simulink model "Regulator_1907_tests_2017a"  (R2017a)
settings: Solver=ode1  StartTime=0.0  StopTime=200  FixedStep=0.01  RelTol=1e-3
values from neighbouring files (symbols this model uses):
  Dist = 0.001    [my_test.m]
  Gain = 0.1    [my_test.m]
  Sat = 0.5    [my_test.m]
  Speed = 3    [my_test.m]
undefined symbols (not defined in the file or in its folder): DiscIntNeverNeededParam
settings Model: Creator=Dmitry  LastModifiedBy=makee
settings OptimizationCC: DefaultUnderspecifiedDataType=single

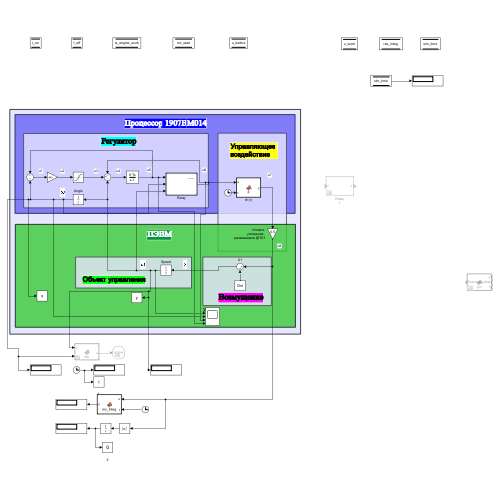
[thumbnail: Simulink's stored preview of the top-level diagram]
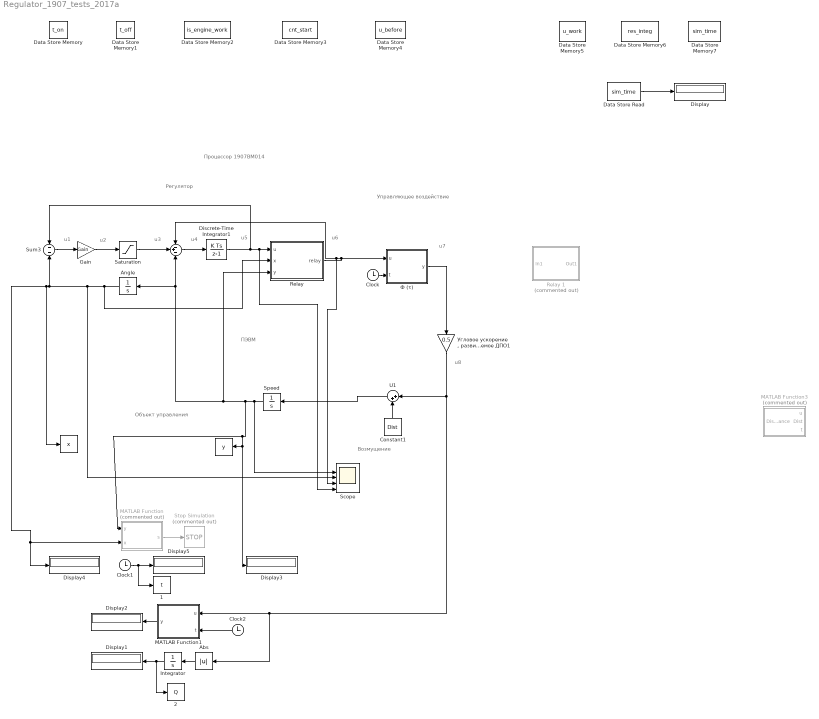
== system Regulator_1907_tests_2017a ==
  note: u8
  note: u7
  note: u6
  note: u5
  note: u4
  note: u3
  note: u2
  note: u1
  note: Объект управления
  note: Управляющее
      | воздействие
  note: Регулятор
  note: Возмущение
  note: ПЭВМ
  note: Процессор 1907ВM014
  " " : ToWorkspace  VariableName=y  SampleTime=-1
  " " : Sum  Inputs=-+-
  " " : ToWorkspace  VariableName=x  SampleTime=-1
  " 1" : ToWorkspace  VariableName=t  SampleTime=-1
  " 2" : ToWorkspace  VariableName=Q  SampleTime=-1
  Abs : Abs
  Angle : Integrator  AbsoluteTolerance=-1
  Clock : Clock
  Clock1 : Clock
  Clock2 : Clock
  Constant1 : Constant  Value=Dist  SampleTime=-1
  Data Store Memory : DataStoreMemory  DataStoreName=t_on  ReadBeforeWriteMsg=warning  WriteAfterWriteMsg=warning  WriteAfterReadMsg=warning  ShowAdditionalParam=off  OutDataTypeStr=double
  Data Store Memory1 : DataStoreMemory  DataStoreName=t_off  ReadBeforeWriteMsg=warning  WriteAfterWriteMsg=warning  WriteAfterReadMsg=warning  ShowAdditionalParam=off  OutDataTypeStr=double
  Data Store Memory2 : DataStoreMemory  DataStoreName=is_engine_work  ReadBeforeWriteMsg=warning  WriteAfterWriteMsg=warning  WriteAfterReadMsg=warning  ShowAdditionalParam=off  OutDataTypeStr=boolean
  Data Store Memory3 : DataStoreMemory  DataStoreName=cnt_start  ReadBeforeWriteMsg=warning  WriteAfterWriteMsg=warning  WriteAfterReadMsg=warning  ShowAdditionalParam=off  OutDataTypeStr=int8
  Data Store Memory4 : DataStoreMemory  DataStoreName=u_before  ReadBeforeWriteMsg=warning  WriteAfterWriteMsg=warning  WriteAfterReadMsg=warning  ShowAdditionalParam=off  OutDataTypeStr=double
  Data Store Memory5 : DataStoreMemory  DataStoreName=u_work  ReadBeforeWriteMsg=warning  WriteAfterWriteMsg=warning  WriteAfterReadMsg=warning  ShowAdditionalParam=off  OutDataTypeStr=double
  Data Store Memory6 : DataStoreMemory  DataStoreName=res_integ  ReadBeforeWriteMsg=warning  WriteAfterWriteMsg=warning  WriteAfterReadMsg=warning  ShowAdditionalParam=off  OutDataTypeStr=double
  Data Store Memory7 : DataStoreMemory  DataStoreName=sim_time  ReadBeforeWriteMsg=warning  WriteAfterWriteMsg=warning  WriteAfterReadMsg=warning  InitialValue=200  ShowAdditionalParam=off  OutDataTypeStr=double
  Data Store Read : DataStoreRead  DataStoreName=sim_time
  Discrete-Time Integrator1 : DiscreteIntegrator  InitialConditionSetting=State (most efficient)  SampleTime=-1  ICPrevOutput=DiscIntNeverNeededParam  ICPrevScaledInput=DiscIntNeverNeededParam
  Display{,1..5} (6 alike) : Display
  Gain : Gain  Gain=Gain
  Integrator : Integrator
  MATLAB Function : MATLAB Function  Commented=on  TreatAsAtomicUnit=on
  MATLAB Function1 : MATLAB Function  TreatAsAtomicUnit=on
  MATLAB Function3 : MATLAB Function  Commented=on  TreatAsAtomicUnit=on
  Relay : MATLAB Function  TreatAsAtomicUnit=on
  Relay 1 : Subsystem  Commented=on
  Saturation : Saturate  UpperLimit=Sat  LowerLimit=-Sat
  Scope : Scope  NumInputPorts=5
  Speed : Integrator  InitialCondition=Speed  AbsoluteTolerance=-1
  Stop Simulation : Stop  Commented=on
  Sum3 : Sum  Inputs=--
  U1 : Sum  Inputs=|++
  "Угловое ускорение, развиваемое ДПО1" : Gain  Gain=0.5
  Ф (τ) : MATLAB Function  TreatAsAtomicUnit=on
  wires:
  Relay/1(relay) -> " "/1, Scope/4, Ф (τ)/1(u)
  Data Store Read/1 -> Display/1
  Angle/1 -> Relay/2(x), " "/1, Display4/1, MATLAB Function/2(x), Sum3/2, Scope/3
  Clock/1 -> Ф (τ)/2(t)
  Sum3/1 -> Gain/1
  Saturation/1 -> " "/2
  Gain/1 -> Saturation/1
  Discrete-Time Integrator1/1 -> Scope/5, Relay/1(u), Sum3/1
  " "/1 -> Discrete-Time Integrator1/1
  Ф (τ)/1(y) -> "Угловое ускорение, развиваемое ДПО1"/1
  Speed/1 -> Scope/2, Display3/1, " "/1, MATLAB Function/1(y), Relay/3(y), " "/3, Angle/1
  Integrator/1 -> " 2"/1, Display1/1
  Abs/1 -> Integrator/1
  "Угловое ускорение, развиваемое ДПО1"/1 -> MATLAB Function1/1(u), Abs/1, U1/1
  Clock2/1 -> MATLAB Function1/2(t)
  MATLAB Function1/1(y) -> Display2/1
  MATLAB Function/1(s) -> Stop Simulation/1
  Clock1/1 -> Display5/1, " 1"/1
  Constant1/1 -> U1/2
  U1/1 -> Speed/1

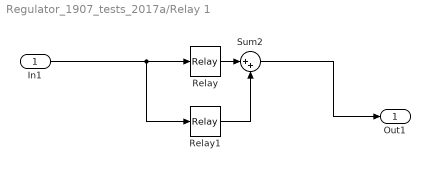
== system Regulator_1907_tests_2017a/Relay 1 ==
  In1 : Inport
  Relay : Relay  OnSwitchValue=0.125  OffSwitchValue=0.125
  Relay1 : Relay  OnSwitchValue=-0.125  OffSwitchValue=-0.125  OnOutputValue=0  OffOutputValue=-1
  Sum2 : Sum  Inputs=|++
  Out1 : Outport
  wires:
  In1/1 -> Relay1/1, Relay/1
  Relay1/1 -> Sum2/2
  Sum2/1 -> Out1/1
  Relay/1 -> Sum2/1

== matlab function Regulator_1907_tests_2017a/MATLAB Function1 ==
  settings: updateMethod=DISCRETE
  data: u input; y output; t input; t_on data_store_memory; t_off data_store_memory; u_work data_store_memory; res_integ data_store_memory; sim_time data_store_memory
function y = my_integ(u, t)
% глобальные переменные
% время включения двигателя
global t_on;
% время выключения двигателя
global t_off;
% Значение сигнала во вермя работы двигателя
global u_work;
% значение результирующего интеграла - суммы
% с каждым импульсом двигателя будет прибавлять площадь прямоугольников
% сюда - это площадь всех прямоугольников на графике u(t) в Scope
% по умолчанию 0
global res_integ;
% Время симуляции системы
global sim_time;

% как только сигнал НЕ нулевой
if u ~= 0
    % Сохраняем его в глобальную переменную
    % - сигнал во время работы двигателя
    u_work = u;
else
    % если сигнал нулевой, то двигатель либо не запускался, либо отработал
    % Если текущее время - это время выключения двигателя
    % И время выключения НЕ равно 0 - значение по умолчанию
    if t == t_off && t_off ~= 0
        % Значит уже точно задали время включения двигателя
        % Тогда можно найти время работы двигателя
        wake_time = t_off - t_on;
        % Время работы двигателя не может быть 0
        % это мы учли в if выше
        % Теперь можно спокойно суммировать с другими площадями
        %  берём абсолюютное значение u_work, иначе площадь будет
        %  отрицательной
        res_integ = res_integ + abs(u_work) * wake_time;
    end
end

% Последняя проверка
% Если  текущее время равно времени окончания симуляции
% и значенеи текущего сигнала - НЕ нулевое
if t == sim_time && u ~= 0
    % нужно добавить последнюю площадь к всем остальным
    % Это случай когда симуляция закончилась на НЕ нулевом сигнале
    % То есть не было задано времени t_off - выключения двигателя
    % назначаем текущее време - временем остановки двигателя
    t_off = t;
    % Найдём время работы двигателя
    wake_time = t_off - t_on;
    % Находим итоговый интеграл
    % Так как текущее значение сигнала u - НЕ нулевое
    % То точно также u_work не равен нулю
    res_integ = res_integ + abs(u_work) * wake_time;
end

% если if в else сработает, то вернёт изменённое значение интеграла
% иначе предыдущее значение
y = res_integ;

== matlab function Regulator_1907_tests_2017a/Ф (τ) ==
  settings: updateMethod=DISCRETE
  data: u input; y output; t input; t_on data_store_memory; t_off data_store_memory; is_engine_work data_store_memory; cnt_start data_store_memory; u_before data_store_memory
% Дополнение импульсов до 30 мс
function y = F(u, t)
% Глобальные переменные, для отслеживания
% включения и выключения двигателя

% Время ВКЛючения двигателя
global t_on;
% Время ВЫКЛючения двигателя
global t_off;
% Логическая переменная (Работает ли двигатель?) - ДА, НЕТ
% По умолчанию - НЕТ - не работает
global is_engine_work;
% Счётчик, сколько раз запускался двигатель
% По умолчанию 0, так как ни разу еще не запускался
global cnt_start;
% Последнее сохраненное значение сигнала
global u_before;

% Проверяем работает ли двигатель
% Если работает
if is_engine_work
    % Находим время работы двигателя
    % Это текущее время минус время запуска двигателя
    wake_time = t - t_on;
    % Если время работы двигателя меньше 30 мс
    if wake_time < 0.03
        % Возвращаем значение сигнала при включении двигателя
        % - это последнее сохранеённое значение сигнала
        y = u_before;
        return
    else
        % Если  время работы двигателя >=30мс
        % Нужно проверить значение сигнала
        % Если значение сигнала не равно сигналу при включении двигателя
        if u ~= u_before
            % Нужно выключить двигатель
            is_engine_work = false;
            % Задаём время выключения двигателя - теущее
            t_off = t;
            % сохранить значение сигнала, ставим именно 0
            % Потому что у нас ступенчатый вид сигнала
            % И должна быть его 0 фаза
            % Не может быть чтобы сигнал был,
            % например 0.5 и сразу стал -0.5
            u_before = 0;
        end
            
        % если if вверху сработает, то выключит двигатель и вернёт 0
        % если if не сработает - то текущий сигнал = сигналу при включении
        % двигателя u_before => Двигатель работает в том же режиме
        % Значит нужно вернуть сигнал, что и при включении двигателя
        % Вернуть значение сигнала
        y = u_before;
        return;
    end
else
    % Двигатель не работает
    % Проверяем запускался ли он хоть раз
    % Если еще не запускался
    if cnt_start == 0
        % То нам не нужно вычислять время спячки двигателя
        % И как только сигнал будет не нулевой
        % Включаем двигатель
        % если текущее значение сигнала НЕ нулевое
        if u ~= 0
            % Включаем двигатель
            is_engine_work = true;
            % Увеличиваем счётчик запусков двигателей
            cnt_start = cnt_start + 1;
            % сохраняем время запуска двигателя - текущее время
            t_on = t;
            % сохранить значение сигнала двигателя при старте
            % - то есть текущее значенеи сигнала
            u_before = u;
        end

        % если if вверху сработает, то вернет сигнал при включении двигателя
        % если не срабоатет, то учитывая, что двигатель еще ни разу не включался
        % то есть u_before = 0, то вернёт 0
        y = u_before;
        return;
    else
        % Двигатель УЖЕ запускался, и нужно отслеживать время спячки двигателя
        % находим время спячки двигателя
        % - это текущее время минус время выключения двигателя
        %sleep_time = t - t_off;
        % Если двигатель спит уже БОЛЬШЕ 200мс
        %if sleep_time > 0.2
            % Нужно проверить значение сигнала
            % Если сигнал НЕ нулевой
            if u ~= 0
                % Включаем двигатель
                is_engine_work = true;
                % Увеличиваем счётчик запусков двигателей
                cnt_start = cnt_start + 1;
                % сохраняем время запуска двигателя - текущее время
                t_on = t;
                % сохранить значение сигнала двигателя при старте
                % - то есть текущее значение сигнала
                u_before = u;
            end
            
            %  Если сработает if вверху - вернёт сигнал при запуске двигателя
            % Если не сработает, то предыдущее сохраненное значение сигнала
            % u_before = 0, и вернёт 0
            % Зачем включать двигатель если он еще спит
            y = u_before;
            return;
       % else
            % Двигатель УЖЕ запускался
            % И спит <= 200мс
            % Значит, ему нужно еще поспать
            % Возвращаем предыдущее значене сигнала
            % Причём u_before = 0
            %y = u_before;
            %return;
        %end
    end
end

== matlab function Regulator_1907_tests_2017a/MATLAB Function ==
  data: y input; s output; x input
function s = fcn(y, x)
% График начинается за пределами прямоугольника
% и только в конце приходит в него
% на основании этого допущения что происходит 
% можно просто смотреть попадают ли точки графика в этот прямоугольник
% если изображающие точки  попадают в заданную прямоугольную область
if (abs(y) <= 0.03 && abs(x) <= 0.125)
    % Завершаем симуляцию
    s = 1;
    return;
else
    % Изображающи точки за пределами прямоугольника стабилизации
    % Продолжаем симуляцию
    s = 0;
    return;
end

== matlab function Regulator_1907_tests_2017a/Relay ==
  data: u input; x input; relay output; y input
function relay = fcn(u, x, y)

    positive = 0.03;
    negative = -0.03;  

  %   При малых углах и угловых скоростях, меняем параметры реле (расширяем область)
  if (abs(y) < 0.03 && abs(x) < 0.125) 
    positive = 0.125;
    negative = -0.125;
  end

  % Преобразуем сигнал либо к -1, либо 0, либо 1
  if (u >= positive) 
    relay = 1;
  elseif (u <= negative) 
    relay = -1;
  else 
    % u принадлежит интервалу (negative, positive )
    relay = 0;
  end

== matlab function Regulator_1907_tests_2017a/MATLAB Function3 ==
  data: u input; Distorbance output; Dist input; t input

%function Distorbance = fcn(u, Dist, x, y,t)
 
% if (abs(y) < 0.03 && abs(x) < 0.125) 
 %   Dist = 0.1 % возмущение в прямоугольнике
  %end
%Distorbance = u + Dist;
%end


function Distorbance = fcn(u, Dist,t)
  if (t > 150) 
    Dist = 0.1 % возмущение в прямоугольнике
  end
Distorbance = u + Dist;
end
